simulink model "Conv_Suspention"  (R2020b)
settings: Solver=VariableStepAuto  StartTime=0.0  StopTime=1  RelTol=1e-3
values from neighbouring files (symbols this model uses):
  Cs = 350    [Suspention.m]
  Ct = 15020    [Suspention.m]
  Ks = 80000    [Suspention.m]
  Kt = 500000    [Suspention.m]
  Ms = 2500    [Suspention.m]
  Mu = 320    [Suspention.m]
settings Model: Creator=sasad  LastModifiedBy=sasad

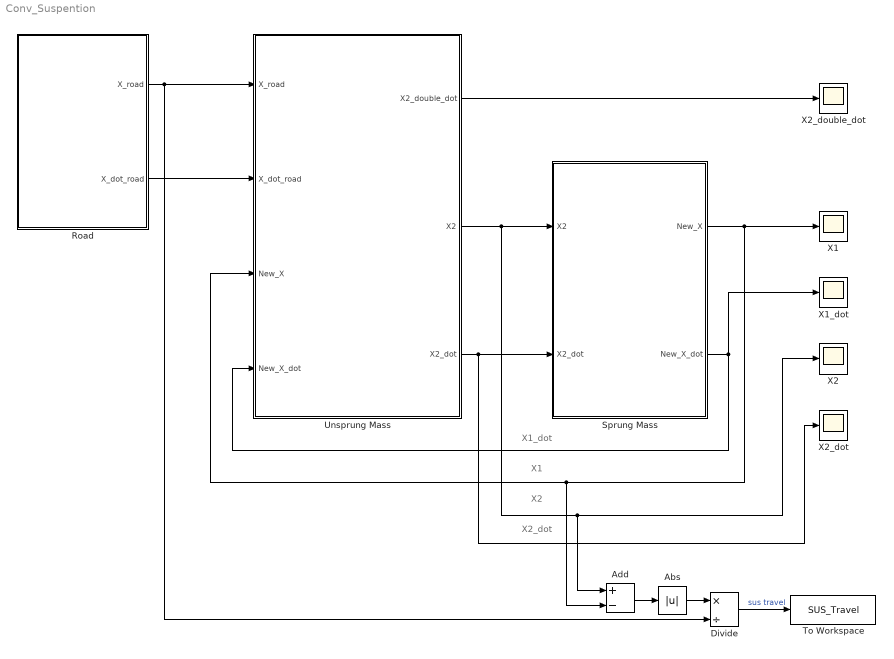
== system Conv_Suspention ==
  note: X1
  note: X2
  note: X1_dot
  note: X2_dot
  Abs : Abs
  Add : Sum  Inputs=+-
  Divide : Product  Inputs=*/
  Road : Subsystem
  Sprung Mass : Subsystem
  To Workspace : ToWorkspace  VariableName=SUS_Travel  SaveFormat=Structure With Time  SampleTime=-1
  Unsprung Mass : Subsystem
  X1 : Scope
  X1_dot : Scope
  X2 : Scope
  X2_dot : Scope
  X2_double_dot : Scope
  wires:
  Unsprung Mass/2(X2) -> X2/1, Add/1, Sprung Mass/1(X2)
  Unsprung Mass/3(X2_dot) -> X2_dot/1, Sprung Mass/2(X2_dot)
  Sprung Mass/2(New_X_dot) -> Unsprung Mass/4(New_X_dot), X1_dot/1
  Sprung Mass/1(New_X) -> X1/1, Add/2, Unsprung Mass/3(New_X)
  Road/1(X_road) -> Divide/2, Unsprung Mass/1(X_road)
  Road/2(X_dot_road) -> Unsprung Mass/2(X_dot_road)
  Unsprung Mass/1(X2_double_dot) -> X2_double_dot/1
  Add/1 -> Abs/1
  Divide/1 -> To Workspace/1  "sus travel"
  Abs/1 -> Divide/1

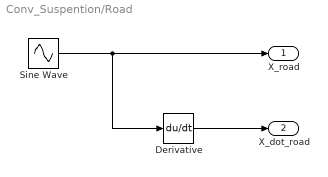
== system Conv_Suspention/Road ==
  Derivative : Derivative
  Sine Wave : Sin  Amplitude=0.02  Bias=1  Frequency=0.05  SampleTime=0
  X_road : Outport
  X_dot_road : Outport  Port=2
  wires:
  Derivative/1 -> X_dot_road/1
  Sine Wave/1 -> X_road/1, Derivative/1

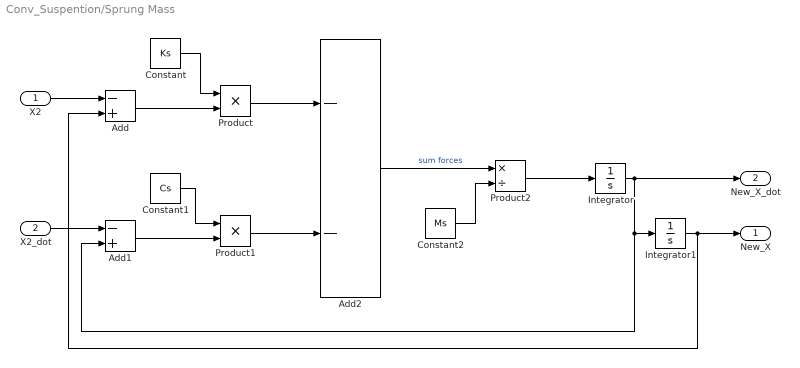
== system Conv_Suspention/Sprung Mass ==
  X2 : Inport
  X2_dot : Inport  Port=2
  Add : Sum  Inputs=-+
  Add1 : Sum  Inputs=-+
  Add2 : Sum  Inputs=--
  Constant : Constant  Value=Ks
  Constant1 : Constant  Value=Cs
  Constant2 : Constant  Value=Ms
  Integrator : Integrator
  Integrator1 : Integrator
  Product : Product
  Product1 : Product
  Product2 : Product  Inputs=*/
  New_X : Outport
  New_X_dot : Outport  Port=2
  wires:
  Add/1 -> Product/2
  X2_dot/1 -> Add1/1
  X2/1 -> Add/1
  Integrator1/1 -> New_X/1, Add/2
  Add1/1 -> Product1/2
  Product/1 -> Add2/1
  Integrator/1 -> New_X_dot/1, Add1/2, Integrator1/1
  Add2/1 -> Product2/1  "sum forces"
  Product1/1 -> Add2/2
  Constant1/1 -> Product1/1
  Constant/1 -> Product/1
  Product2/1 -> Integrator/1
  Constant2/1 -> Product2/2

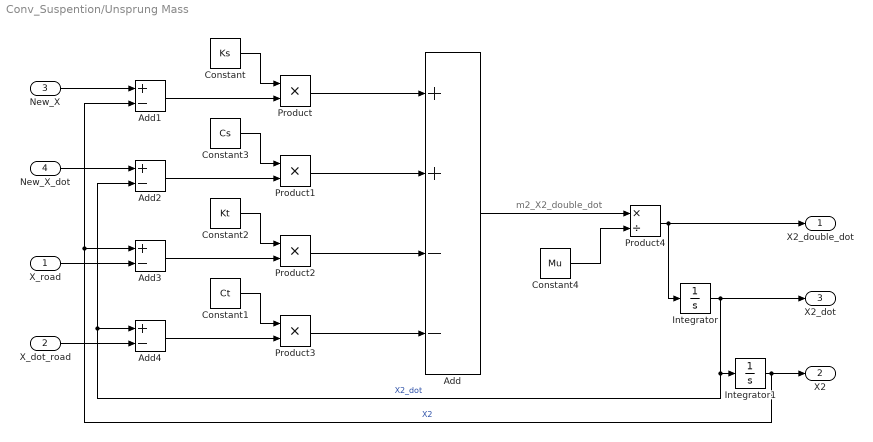
== system Conv_Suspention/Unsprung Mass ==
  note: m2_X2_double_dot
  X_road : Inport
  X_dot_road : Inport  Port=2
  New_X : Inport  Port=3
  New_X_dot : Inport  Port=4
  Add : Sum  Inputs=++--
  Add{1..4} (4 alike) : Sum  Inputs=+-
  Constant : Constant  Value=Ks
  Constant1 : Constant  Value=Ct
  Constant2 : Constant  Value=Kt
  Constant3 : Constant  Value=Cs
  Constant4 : Constant  Value=Mu
  Integrator : Integrator
  Integrator1 : Integrator
  Product{,1..3} (4 alike) : Product
  Product4 : Product  Inputs=*/
  X2_double_dot : Outport
  X2 : Outport  Port=2
  X2_dot : Outport  Port=3
  wires:
  Integrator1/1 -> X2/1, Add1/2, Add3/1  "X2"
  Constant3/1 -> Product1/1
  Integrator/1 -> X2_dot/1, Add2/2, Add4/1, Integrator1/1  "X2_dot"
  Product/1 -> Add/1
  Product2/1 -> Add/3
  Add/1 -> Product4/1
  Constant/1 -> Product/1
  Constant1/1 -> Product3/1
  Product3/1 -> Add/4
  New_X_dot/1 -> Add2/1
  New_X/1 -> Add1/1
  Add1/1 -> Product/2
  X_road/1 -> Add3/2
  Add4/1 -> Product3/2
  Add3/1 -> Product2/2
  Constant4/1 -> Product4/2
  Product4/1 -> X2_double_dot/1, Integrator/1
  Constant2/1 -> Product2/1
  Product1/1 -> Add/2
  Add2/1 -> Product1/2
  X_dot_road/1 -> Add4/2
